simulink model "D53_LKAS_JLU_20200903_0931"  (R2018b)
settings: Solver=ode3  StartTime=0.0  StopTime=10.0  FixedStep=0.01  RelTol=1e-3  EnableMultiTasking=on
model workspace (MAT data in the model file):
  MCOS : class17 (value not decoded)
  MCOS : class17 (value not decoded)
  MCOS : class17 (value not decoded)
  MCOS : class17 (value not decoded)
  MCOS : class17 (value not decoded)
  MCOS : class17 (value not decoded)
  MCOS : class17 (value not decoded)
  MCOS : class17 (value not decoded)
  MCOS : class17 (value not decoded)
  MCOS : class17 (value not decoded)
  MCOS : class17 (value not decoded)
  MCOS : class17 (value not decoded)
  MCOS : class17 (value not decoded)
  MCOS : class17 (value not decoded)
  MCOS : class17 (value not decoded)
  MCOS : class17 (value not decoded)
  MCOS : class17 (value not decoded)
  MCOS : class17 (value not decoded)
  MCOS : class17 (value not decoded)
  MCOS : class17 (value not decoded)
  MCOS : class17 (value not decoded)
  MCOS : class17 (value not decoded)
  MCOS : class17 (value not decoded)
  MCOS : class17 (value not decoded)
  MCOS : class17 (value not decoded)
  MCOS : class17 (value not decoded)
  MCOS : class17 (value not decoded)
  MCOS : class17 (value not decoded)
  MCOS : class17 (value not decoded)
  MCOS : class17 (value not decoded)
  MCOS : class17 (value not decoded)
  MCOS : class17 (value not decoded)
  MCOS : class17 (value not decoded)
  MCOS : class17 (value not decoded)
  MCOS : class17 (value not decoded)
  MCOS : class17 (value not decoded)
  MCOS : class17 (value not decoded)
  MCOS : class17 (value not decoded)
  MCOS : class17 (value not decoded)
  MCOS : class17 (value not decoded)
  MCOS : class17 (value not decoded)
  MCOS : class17 (value not decoded)
  MCOS : class17 (value not decoded)
  MCOS : class17 (value not decoded)
  MCOS : class17 (value not decoded)
  MCOS : class17 (value not decoded)
  MCOS : class17 (value not decoded)
  MCOS : class17 (value not decoded)
  MCOS : class17 (value not decoded)
  MCOS : class17 (value not decoded)
  MCOS : class17 (value not decoded)
  MCOS : class17 (value not decoded)
  MCOS : class17 (value not decoded)
  MCOS : class17 (value not decoded)
  MCOS : class17 (value not decoded)
  MCOS : class17 (value not decoded)
  MCOS : class17 (value not decoded)
  MCOS : class17 (value not decoded)
  MCOS : class17 (value not decoded)
  MCOS : class17 (value not decoded)
  MCOS : class17 (value not decoded)
  MCOS : class17 (value not decoded)
  MCOS : class17 (value not decoded)
  MCOS : class17 (value not decoded)
  MCOS : class17 (value not decoded)
  MCOS : class17 (value not decoded)
  MCOS : class17 (value not decoded)
  MCOS : class17 (value not decoded)
  MCOS : class17 (value not decoded)
  MCOS : class17 (value not decoded)
  MCOS : class17 (value not decoded)
  MCOS : class17 (value not decoded)
  MCOS : class17 (value not decoded)
  MCOS : class17 (value not decoded)
  MCOS : class17 (value not decoded)
  MCOS : class17 (value not decoded)
  MCOS : class17 (value not decoded)
  MCOS : class17 (value not decoded)
  MCOS : class17 (value not decoded)
  MCOS : class17 (value not decoded)
  MCOS : class17 (value not decoded)
  MCOS : class17 (value not decoded)
  MCOS : class17 (value not decoded)
  MCOS : class17 (value not decoded)
  MCOS : class17 (value not decoded)
  MCOS : class17 (value not decoded)
  MCOS : class17 (value not decoded)
  MCOS : class17 (value not decoded)
  MCOS : class17 (value not decoded)
undefined symbols (not defined in the file): LKA_CarWidth, LKA_SampleTime, LKA_StrRatio_C, LKA_Veh2CamL_C, LKA_Veh2CamW_C, LKA_WhlBaseL_C, LL_CompSWA_C, LL_CrvtPrvwT_C, LL_DesDvt_C, LL_DvtComp_C, LL_DvtPrvwT_C, LL_DvtSpdDet_vDvtSpdMin_C, LL_HdAgExT_C, LL_HdAgPrvwT_C, LL_LAccMax_C, LL_LAccRMax_C, LL_LDW_EarliestWarnLine_C, LL_LDW_LatestWarnLine_C, LL_LDWS_SUPPRESS_HEADING, LL_LFClb_TFC_DiffCtlBalance, LL_LFClb_TFC_DiffCtrlMaxSWA, LL_LFClb_TFC_DiffCtrlRatio, LL_LFClb_TFC_facmGainLutGain1_C, LL_LFClb_TFC_facmGainLutGain2_C, LL_LFClb_TFC_facmIntegRatio, LL_LFClb_TFC_facmKlat_C, LL_LFClb_TFC_FfCtlRatio_C, LL_LFClb_TFC_phiIntegCtlMaxSWA_C, LL_LFClb_TFC_tiKlatPrvwT_C, LL_LFClb_TFC_vGainLutVehSpdLwr_C, LL_LFClb_TFC_vGainLutVehSpdUpr_C, LL_LKA_EarliestWarnLine_C, LL_LKA_LatestWarnLine_C, LL_LKAExPrcs_ExitC0Dvt, LL_LKAExPrcs_ExitC0Swt, LL_LKAExPrcs_tiExitTime1, LL_LKAExPrcs_tiExitTime2, LL_LKAExPrcs_tiExitTime3, LL_LKAS_OUT_OF_CONTROL_LAT_VEL, LL_LKAS_OUT_OF_CONTROL_TTLC, LL_LKASWASyn_M0, LL_LKASWASyn_M1, LL_LKASWASyn_M2, LL_LKASWASyn_M3K, LL_LKASWASyn_SWAaddMax, LL_LKASWASyn_T2, LL_LKASWASyn_tiTrqSwaRtTime, LL_LKASWASyn_tiTrqSwaTime, LL_LKASWASyn_TrqMax, LL_LKASWASyn_TrqSwaAddSwt, LL_LKASWASyn_TrqSwaRateDiff, LL_LSpdCompT_C, LL_lStpLngth_C, LL_MAX_DELAY_EPSSTAR_TIME, LL_MAX_DRIVER_TORQUE_DISABLE, LL_MAX_DRIVER_TORQUE_ENABLE, LL_MAX_LANE_WIDTH_DISABLE, LL_MAX_LANE_WIDTH_ENABLE, LL_MAX_LAT_ACC_DISABLE, LL_MAX_LAT_ACC_ENABLE ... (+30)
libraries: simulink x135, canmsglib x41, dspstat3 x3, simulink_extras x1
(part 6 of 18)

== system D53_LKAS_JLU_20200903_0931/SignalBusCreator/Subsystem3 ==
  Bus Creator20 : BusCreator  Inputs=10
  CAN Receive (CANRX) : S-Function  FunctionName=CAN_Rec_P  Parameters=uint8(Module-1),uint32(ID),uint8(Frameformat-1),uint8(Newflag),uint8(FIFO),double(sampletime)  SFunctionDeploymentMode=off  EnableBusSupport=off  mask(CAN_receive){Module=CAN_2, ID=1531, Frameformat=Extended (29-bit identifier), Newflag=off, FIFO=off, sampletime=0.01}
      mask prompts: Module "CAN Port:"; ID "CAN Frame ID:"; Frameformat "CAN Frame Format:"; FIFO "Overflow flag"
      mask init:
      | maskdisplay = canrecicon(Module,ID,Frameformat,Newflag,FIFO);
      | set_param(gcb, 'MaskDisplay', maskdisplay);
      mask TypeOptions Module: CAN_0 | CAN_1 | CAN_2 | CAN_3
      mask TypeOptions Frameformat: Standard (11-bit identifier) | Extended (29-bit identifier)
      mask Display: color('blue');text(0.98,0.9,'MPC5675K','horizontalAlignment','right');color('black');text(0.5,0.6,'FlexCAN_2 Receive','horizontalAlignment','center');text(0.5,0.35,'Extended ID:1531','horizontalAlignment','center');port_label('output',1,'CAN_Msg');
  CAN Receive (CANRX)1 : S-Function  FunctionName=CAN_Rec_P  Parameters=uint8(Module-1),uint32(ID),uint8(Frameformat-1),uint8(Newflag),uint8(FIFO),double(sampletime)  SFunctionDeploymentMode=off  EnableBusSupport=off  mask(CAN_receive){Module=CAN_2, ID=1523, Frameformat=Extended (29-bit identifier), Newflag=off, FIFO=off, sampletime=0.01}
      mask prompts: Module "CAN Port:"; ID "CAN Frame ID:"; Frameformat "CAN Frame Format:"; FIFO "Overflow flag"
      mask init:
      | maskdisplay = canrecicon(Module,ID,Frameformat,Newflag,FIFO);
      | set_param(gcb, 'MaskDisplay', maskdisplay);
      mask TypeOptions Module: CAN_0 | CAN_1 | CAN_2 | CAN_3
      mask TypeOptions Frameformat: Standard (11-bit identifier) | Extended (29-bit identifier)
      mask Display: color('blue');text(0.98,0.9,'MPC5675K','horizontalAlignment','right');color('black');text(0.5,0.6,'FlexCAN_2 Receive','horizontalAlignment','center');text(0.5,0.35,'Extended ID:1523','horizontalAlignment','center');port_label('output',1,'CAN_Msg');
  CAN Unpack1 : canmsglib/CAN Unpack  CANdbFile=D:\Work\02_LKA\LKAS\Documents\D53-SensorCAN.dbc  MsgList=Video_Lane_Next_Left_B  MsgName=Video_Lane_Next_Left_B  MsgIDType=Standard (11-bit identifier)  MsgIdentifier=1523  MsgLength=4  SignalInfo=Line_Width_5F3$17$7$2$2$1$0$1.000000e-02$0$0$1.270000e+00$#Me_Line_Changed_5F3$16$1$2$2$1$0$1$0$0$1$#TLC_5F3$8$8$2$2$1$0$1.000000e-02$0$0$2.550000e+00$#View_Range_5F3$0$8$2$2$1$0$5.000000e-01$0$0$1.275000e+02$#  NSignals=4  IDPort=off  TimestampPort=off  ErrorPort=off  RemotePort=off  LengthPort=off  StatusPort=off  StartBits=str2num('[int32(17);int32(16);int32(8);int32(0)]')  SignalSizes=str2num('[int32(7);int32(1);int32(8);int32(8)]')  ByteOrders=str2num('[int32(2);int32(2);int32(2);int32(2)]')  DataTypes=str2num('[int32(2);int32(2);int32(2);int32(2)]')  MultiplexTypes=str2num('[int32(1);int32(1);int32(1);int32(1)]')  MultiplexValues=str2num('[double(0);double(0);double(0);double(0)]')  Factors=str2num('[double(1.000000e-02);double(1);double(1.000000e-02);double(5.000000e-01)]')  Offsets=str2num('[double(0);double(0);double(0);double(0)]')  Minimums=str2num('[double(0);double(0);double(0);double(0)]')  Maximums=str2num('[double(1.270000e+00);double(1);double(2.550000e+00);double(1.275000e+02)]')  ApplyMinMax=off
      settings: SourceProductName=Simulink Real-Time  SourceProductBaseCode=XP  DataFormat=CANdb specified signals
  CAN Unpack13 : canmsglib/CAN Unpack  CANdbFile=D:\Work\02_LKA\LKAS\Documents\D53-SensorCAN.dbc  MsgList=Video_Lane_Next_Left_A  MsgName=Video_Lane_Next_Left_A  MsgIDType=Standard (11-bit identifier)  MsgIdentifier=1531  MsgLength=8  SignalInfo=C0_5FB$44$12$2$1$1$0$1.000000e-02$0$-2.048000e+01$2.047000e+01$#C1_5FB$50$10$2$1$1$0$9.765625e-04$0$-3.570000e-01$3.570000e-01$#C2_5FB$24$16$2$1$1$0$1.000000e-06$0$-3.276800e-02$3.276600e-02$#C3_5FB$8$16$2$1$1$0$4.000000e-09$0$-1.310720e-04$1.310680e-04$#Line_Type_5FB$59$3$2$2$1$0$1$0$0$7$#Quality_5FB$62$2$2$2$1$0$1$0$0$3$#  NSignals=6  IDPort=off  TimestampPort=off  ErrorPort=off  RemotePort=off  LengthPort=off  StatusPort=off  StartBits=str2num('[int32(44);int32(50);int32(24);int32(8);int32(59);int32(62)]')  SignalSizes=str2num('[int32(12);int32(10);int32(16);int32(16);int32(3);int32(2)]')  ByteOrders=str2num('[int32(2);int32(2);int32(2);int32(2);int32(2);int32(2)]')  DataTypes=str2num('[int32(1);int32(1);int32(1);int32(1);int32(2);int32(2)]')  MultiplexTypes=str2num('[int32(1);int32(1);int32(1);int32(1);int32(1);int32(1)]')  MultiplexValues=str2num('[double(0);double(0);double(0);double(0);double(0);double(0)]')  Factors=str2num('[double(1.000000e-02);double(9.765625e-04);double(1.000000e-06);double(4.000000e-09);double(1);double(1)]')  Offsets=str2num('[double(0);double(0);double(0);double(0);double(0);double(0)]')  Minimums=str2num('[double(-2.048000e+01);double(-3.570000e-01);double(-3.276800e-02);double(-1.310720e-04);double(0);double(0)]')  Maximums=str2num('[double(2.047000e+01);double(3.570000e-01);double(3.276600e-02);double(1.310680e-04);double(7);double(3)]')  ApplyMinMax=off
      settings: SourceProductName=Simulink Real-Time  SourceProductBaseCode=XP  DataFormat=CANdb specified signals
  Data Type Conversion{,1..3,5..6,9} (7 alike) : DataTypeConversion  OutDataTypeStr=single
  Data Type Conversion4 : DataTypeConversion  OutDataTypeStr=uint8
  Data Type Conversion7 : DataTypeConversion  OutDataTypeStr=uint8
  Data Type Conversion8 : DataTypeConversion  OutDataTypeStr=uint8
  bsOriL1Info : Outport
  wires:
  CAN Receive (CANRX)/1 -> CAN Unpack13/1
  Data Type Conversion/1 -> Bus Creator20/4  "O_L1_C0"
  CAN Unpack13/4 -> Data Type Conversion3/1
  CAN Unpack13/5 -> Data Type Conversion7/1
  Data Type Conversion6/1 -> Bus Creator20/9  "O_L1_W"
  CAN Unpack13/2 -> Data Type Conversion1/1
  CAN Unpack1/4 -> Data Type Conversion5/1
  Data Type Conversion4/1 -> Bus Creator20/5  "O_L1_Q"
  CAN Unpack1/2 -> Data Type Conversion8/1
  CAN Unpack13/6 -> Data Type Conversion4/1
  CAN Unpack13/1 -> Data Type Conversion/1
  CAN Unpack1/1 -> Data Type Conversion6/1
  CAN Unpack1/3 -> Data Type Conversion9/1
  CAN Unpack13/3 -> Data Type Conversion2/1
  Data Type Conversion9/1 -> Bus Creator20/8  "O_L1_TLC"
  Data Type Conversion7/1 -> Bus Creator20/6  "O_L1_Type"
  Bus Creator20/1 -> bsOriL1Info/1  "bsOriL1Info"
  Data Type Conversion5/1 -> Bus Creator20/7  "O_L1_VR"
  Data Type Conversion3/1 -> Bus Creator20/1  "O_L1_C3"
  Data Type Conversion8/1 -> Bus Creator20/10  "O_L1_LC"
  Data Type Conversion1/1 -> Bus Creator20/3  "O_L1_C1"
  Data Type Conversion2/1 -> Bus Creator20/2  "O_L1_C2"
  CAN Receive (CANRX)1/1 -> CAN Unpack1/1

== system D53_LKAS_JLU_20200903_0931/SignalBusCreator/Subsystem4 ==
  Bus Creator22 : BusCreator  Inputs=10
  CAN Receive (CANRX) : S-Function  FunctionName=CAN_Rec_P  Parameters=uint8(Module-1),uint32(ID),uint8(Frameformat-1),uint8(Newflag),uint8(FIFO),double(sampletime)  SFunctionDeploymentMode=off  EnableBusSupport=off  mask(CAN_receive){Module=CAN_2, ID=1534, Frameformat=Extended (29-bit identifier), Newflag=off, FIFO=off, sampletime=0.01}
      mask prompts: Module "CAN Port:"; ID "CAN Frame ID:"; Frameformat "CAN Frame Format:"; FIFO "Overflow flag"
      mask init:
      | maskdisplay = canrecicon(Module,ID,Frameformat,Newflag,FIFO);
      | set_param(gcb, 'MaskDisplay', maskdisplay);
      mask TypeOptions Module: CAN_0 | CAN_1 | CAN_2 | CAN_3
      mask TypeOptions Frameformat: Standard (11-bit identifier) | Extended (29-bit identifier)
      mask Display: color('blue');text(0.98,0.9,'MPC5675K','horizontalAlignment','right');color('black');text(0.5,0.6,'FlexCAN_2 Receive','horizontalAlignment','center');text(0.5,0.35,'Extended ID:1534','horizontalAlignment','center');port_label('output',1,'CAN_Msg');
  CAN Receive (CANRX)1 : S-Function  FunctionName=CAN_Rec_P  Parameters=uint8(Module-1),uint32(ID),uint8(Frameformat-1),uint8(Newflag),uint8(FIFO),double(sampletime)  SFunctionDeploymentMode=off  EnableBusSupport=off  mask(CAN_receive){Module=CAN_2, ID=1524, Frameformat=Extended (29-bit identifier), Newflag=off, FIFO=off, sampletime=0.01}
      mask prompts: Module "CAN Port:"; ID "CAN Frame ID:"; Frameformat "CAN Frame Format:"; FIFO "Overflow flag"
      mask init:
      | maskdisplay = canrecicon(Module,ID,Frameformat,Newflag,FIFO);
      | set_param(gcb, 'MaskDisplay', maskdisplay);
      mask TypeOptions Module: CAN_0 | CAN_1 | CAN_2 | CAN_3
      mask TypeOptions Frameformat: Standard (11-bit identifier) | Extended (29-bit identifier)
      mask Display: color('blue');text(0.98,0.9,'MPC5675K','horizontalAlignment','right');color('black');text(0.5,0.6,'FlexCAN_2 Receive','horizontalAlignment','center');text(0.5,0.35,'Extended ID:1524','horizontalAlignment','center');port_label('output',1,'CAN_Msg');
  CAN Unpack1 : canmsglib/CAN Unpack  CANdbFile=D:\Work\02_LKA\LKAS\Documents\D53-SensorCAN.dbc  MsgList=Video_Lane_Next_Right_B  MsgName=Video_Lane_Next_Right_B  MsgIDType=Standard (11-bit identifier)  MsgIdentifier=1524  MsgLength=4  SignalInfo=Line_Width_5F4$17$7$2$2$1$0$1.000000e-02$0$0$1.270000e+00$#Me_Line_Changed_5F4$16$1$2$2$1$0$1$0$0$1$#TLC_5F4$8$8$2$2$1$0$1.000000e-02$0$0$2.550000e+00$#View_Range_5F4$0$8$2$2$1$0$5.000000e-01$0$0$1.275000e+02$#  NSignals=4  IDPort=off  TimestampPort=off  ErrorPort=off  RemotePort=off  LengthPort=off  StatusPort=off  StartBits=str2num('[int32(17);int32(16);int32(8);int32(0)]')  SignalSizes=str2num('[int32(7);int32(1);int32(8);int32(8)]')  ByteOrders=str2num('[int32(2);int32(2);int32(2);int32(2)]')  DataTypes=str2num('[int32(2);int32(2);int32(2);int32(2)]')  MultiplexTypes=str2num('[int32(1);int32(1);int32(1);int32(1)]')  MultiplexValues=str2num('[double(0);double(0);double(0);double(0)]')  Factors=str2num('[double(1.000000e-02);double(1);double(1.000000e-02);double(5.000000e-01)]')  Offsets=str2num('[double(0);double(0);double(0);double(0)]')  Minimums=str2num('[double(0);double(0);double(0);double(0)]')  Maximums=str2num('[double(1.270000e+00);double(1);double(2.550000e+00);double(1.275000e+02)]')  ApplyMinMax=off
      settings: SourceProductName=Simulink Real-Time  SourceProductBaseCode=XP  DataFormat=CANdb specified signals
  CAN Unpack13 : canmsglib/CAN Unpack  CANdbFile=D:\Work\02_LKA\LKAS\Documents\D53-SensorCAN.dbc  MsgList=Video_Lane_Next_Right_A  MsgName=Video_Lane_Next_Right_A  MsgIDType=Standard (11-bit identifier)  MsgIdentifier=1534  MsgLength=8  SignalInfo=C0_5FE$44$12$2$1$1$0$1.000000e-02$0$-2.048000e+01$2.047000e+01$#C1_5FE$50$10$2$1$1$0$9.765625e-04$0$-3.570000e-01$3.570000e-01$#C2_5FE$24$16$2$1$1$0$1.000000e-06$0$-3.276800e-02$3.276600e-02$#C3_5FE$8$16$2$1$1$0$4.000000e-09$0$-1.310720e-04$1.310680e-04$#Line_Type_5FE$59$3$2$2$1$0$1$0$0$7$#Quality_5FE$62$2$2$2$1$0$1$0$0$3$#  NSignals=6  IDPort=off  TimestampPort=off  ErrorPort=off  RemotePort=off  LengthPort=off  StatusPort=off  StartBits=str2num('[int32(44);int32(50);int32(24);int32(8);int32(59);int32(62)]')  SignalSizes=str2num('[int32(12);int32(10);int32(16);int32(16);int32(3);int32(2)]')  ByteOrders=str2num('[int32(2);int32(2);int32(2);int32(2);int32(2);int32(2)]')  DataTypes=str2num('[int32(1);int32(1);int32(1);int32(1);int32(2);int32(2)]')  MultiplexTypes=str2num('[int32(1);int32(1);int32(1);int32(1);int32(1);int32(1)]')  MultiplexValues=str2num('[double(0);double(0);double(0);double(0);double(0);double(0)]')  Factors=str2num('[double(1.000000e-02);double(9.765625e-04);double(1.000000e-06);double(4.000000e-09);double(1);double(1)]')  Offsets=str2num('[double(0);double(0);double(0);double(0);double(0);double(0)]')  Minimums=str2num('[double(-2.048000e+01);double(-3.570000e-01);double(-3.276800e-02);double(-1.310720e-04);double(0);double(0)]')  Maximums=str2num('[double(2.047000e+01);double(3.570000e-01);double(3.276600e-02);double(1.310680e-04);double(7);double(3)]')  ApplyMinMax=off
      settings: SourceProductName=Simulink Real-Time  SourceProductBaseCode=XP  DataFormat=CANdb specified signals
  Data Type Conversion{,6..8,10..11,14} (7 alike) : DataTypeConversion  OutDataTypeStr=single
  Data Type Conversion12 : DataTypeConversion  OutDataTypeStr=uint8
  Data Type Conversion13 : DataTypeConversion  OutDataTypeStr=uint8
  Data Type Conversion9 : DataTypeConversion  OutDataTypeStr=uint8
  bsOriR1Info : Outport
  wires:
  Data Type Conversion6/1 -> Bus Creator22/3  "O_R1_C1"
  Data Type Conversion11/1 -> Bus Creator22/9  "O_R1_W"
  Data Type Conversion14/1 -> Bus Creator22/8  "O_R1_TLC"
  Data Type Conversion/1 -> Bus Creator22/4  "O_R1_C0"
  Data Type Conversion7/1 -> Bus Creator22/2  "O_R1_C2"
  Data Type Conversion9/1 -> Bus Creator22/5  "O_R1_Q"
  Data Type Conversion13/1 -> Bus Creator22/10  "O_R1_LC"
  Data Type Conversion8/1 -> Bus Creator22/1  "O_R1_C3"
  CAN Unpack13/2 -> Data Type Conversion6/1
  CAN Unpack13/3 -> Data Type Conversion7/1
  Data Type Conversion12/1 -> Bus Creator22/6  "O_R1_Type"
  Data Type Conversion10/1 -> Bus Creator22/7  "O_R1_VR"
  CAN Unpack13/1 -> Data Type Conversion/1
  CAN Unpack1/4 -> Data Type Conversion10/1
  CAN Receive (CANRX)/1 -> CAN Unpack13/1
  CAN Unpack1/3 -> Data Type Conversion14/1
  CAN Unpack13/5 -> Data Type Conversion12/1
  CAN Unpack13/6 -> Data Type Conversion9/1
  CAN Unpack1/2 -> Data Type Conversion13/1
  CAN Unpack1/1 -> Data Type Conversion11/1
  CAN Unpack13/4 -> Data Type Conversion8/1
  Bus Creator22/1 -> bsOriR1Info/1  "bsOriR1Info"
  CAN Receive (CANRX)1/1 -> CAN Unpack1/1

== system D53_LKAS_JLU_20200903_0931/SignalBusCreator/Subsystem5 ==
  Bus Creator3 : BusCreator  Inputs=4
  CAN Recv (CANRx]) : S-Function  FunctionName=CAN_Rec_P  Parameters=uint8(Module-1),uint32(ID),uint8(Frameformat-1),uint8(Newflag),uint8(FIFO),double(sampletime)  SFunctionDeploymentMode=off  EnableBusSupport=off  mask(CAN_receive){Module=CAN_1, ID=773, Frameformat=Standard (11-bit identifier), Newflag=off, FIFO=off, sampletime=0.01}
      mask prompts: Module "CAN Port:"; ID "CAN Frame ID:"; Frameformat "CAN Frame Format:"; FIFO "Overflow flag"
      mask init:
      | maskdisplay = canrecicon(Module,ID,Frameformat,Newflag,FIFO);
      | set_param(gcb, 'MaskDisplay', maskdisplay);
      mask TypeOptions Module: CAN_0 | CAN_1 | CAN_2 | CAN_3
      mask TypeOptions Frameformat: Standard (11-bit identifier) | Extended (29-bit identifier)
      mask Display: color('blue');text(0.98,0.9,'MPC5675K','horizontalAlignment','right');color('black');text(0.5,0.6,'FlexCAN_1 Receive','horizontalAlignment','center');text(0.5,0.35,'Standard ID:773','horizontalAlignment','center');port_label('output',1,'CAN_Msg');
  CAN Unpack1 : canmsglib/CAN Unpack  CANdbFile=D:\Work\02_LKA\LKAS\Documents\D53-PSA1CAN.dbc  MsgList=EPS_305_PSA1  MsgName=EPS_305_PSA1  MsgIDType=Standard (11-bit identifier)  MsgIdentifier=773  MsgLength=7  SignalInfo=Absolute_Steering_Wheel_angle$54$1$2$2$1$0$1$0$-Inf$Inf$#Initialization_steering_angle$55$1$2$2$1$0$1$0$-Inf$Inf$#Internal_SWS_status$24$1$2$2$1$0$1$0$-Inf$Inf$#SWS_calibration$25$1$2$2$1$0$1$0$-Inf$Inf$#SWS_checksum$36$4$2$2$1$0$1$0$-Inf$Inf$#SWS_fault_code$27$4$2$2$1$0$1$0$-Inf$Inf$#SWS_trim$26$1$2$2$1$0$1$0$-Inf$Inf$#Steering_wheel_angle$8$16$2$1$1$0$1.000000e-01$0$-780$780$#Steering_wheel_rotation_speed$16$8$2$2$1$0$4$0$0$1016$#Steering_wheel_sensor_direction$31$1$2$2$1$0$1$0$-Inf$Inf$#bits_Compute_counter_for_SWS$32$4$2$2$1$0$1$0$0$15$#indication_of_steering_wheel$52$2$2$2$1$0$1$0$-Inf$Inf$#  NSignals=12  IDPort=off  TimestampPort=off  ErrorPort=off  RemotePort=off  LengthPort=off  StatusPort=off  StartBits=str2num('[int32(54);int32(55);int32(24);int32(25);int32(36);int32(27);int32(26);int32(8);int32(16);int32(31);int32(32);int32(52)]')  SignalSizes=str2num('[int32(1);int32(1);int32(1);int32(1);int32(4);int32(4);int32(1);int32(16);int32(8);int32(1);int32(4);int32(2)]')  ByteOrders=str2num('[int32(2);int32(2);int32(2);int32(2);int32(2);int32(2);int32(2);int32(2);int32(2);int32(2);int32(2);int32(2)]')  DataTypes=str2num('[int32(2);int32(2);int32(2);int32(2);int32(2);int32(2);int32(2);int32(1);int32(2);int32(2);int32(2);int32(2)]')  MultiplexTypes=str2num('[int32(1);int32(1);int32(1);int32(1);int32(1);int32(1);int32(1);int32(1);int32(1);int32(1);int32(1);int32(1)]')  MultiplexValues=str2num('[double(0);double(0);double(0);double(0);double(0);double(0);double(0);double(0);double(0);double(0);double(0);double(0)]')  Factors=str2num('[double(1);double(1);double(1);double(1);double(1);double(1);double(1);double(1.000000e-01);double(4);double(1);double(1);double(1)]')  Offsets=str2num('[double(0);double(0);double(0);double(0);double(0);double(0);double(0);double(0);double(0);double(0);double(0);double(0)]')  Minimums=str2num('[double(-Inf);double(-Inf);double(-Inf);double(-Inf);double(-Inf);double(-Inf);double(-Inf);double(-780);double(0);double(-Inf);double(0);double(-Inf)]')  Maximums=str2num('[double(Inf);double(Inf);double(Inf);double(Inf);double(Inf);double(Inf);double(Inf);double(780);double(1016);double(Inf);double(15);double(Inf)]')  ApplyMinMax=off
      settings: SourceProductName=Simulink Real-Time  SourceProductBaseCode=XP  DataFormat=CANdb specified signals
  Data Type Conversion1 : DataTypeConversion  OutDataTypeStr=single
  Data Type Conversion2 : DataTypeConversion  OutDataTypeStr=single
  Data Type Conversion46 : DataTypeConversion  OutDataTypeStr=uint8
  Data Type Conversion47 : DataTypeConversion  OutDataTypeStr=uint8
  Terminator{1..8} (8 alike) : Terminator
  bsSWAInfo : Outport
  wires:
  Data Type Conversion46/1 -> Bus Creator3/3  "SWS_Fault_Code"
  CAN Unpack1/4 -> Terminator3/1
  CAN Unpack1/5 -> Terminator4/1
  CAN Unpack1/11 -> Terminator7/1
  Bus Creator3/1 -> bsSWAInfo/1  "bsSWAInfo"
  CAN Unpack1/12 -> Terminator8/1
  CAN Unpack1/8 -> Data Type Conversion1/1  "SWARx_phiSWA"
  CAN Unpack1/2 -> Terminator2/1  "SWARx_phiSWA"
  CAN Unpack1/9 -> Data Type Conversion2/1  "SW_Angle_Speed"
  CAN Unpack1/10 -> Terminator6/1
  CAN Unpack1/6 -> Data Type Conversion46/1
  CAN Unpack1/3 -> Data Type Conversion47/1
  CAN Recv (CANRx])/1 -> CAN Unpack1/1
  Data Type Conversion47/1 -> Bus Creator3/4  "SAS_In_Status"
  CAN Unpack1/1 -> Terminator1/1
  CAN Unpack1/7 -> Terminator5/1
  Data Type Conversion1/1 -> Bus Creator3/1  "SW_Angle"
  Data Type Conversion2/1 -> Bus Creator3/2  "SW_Angle_Speed"

== system D53_LKAS_JLU_20200903_0931/SignalBusCreator/Subsystem6 ==
  Bus Creator2 : BusCreator  Inputs=9
  CAN Recv : S-Function  FunctionName=CAN_Rec_P  Parameters=uint8(Module-1),uint32(ID),uint8(Frameformat-1),uint8(Newflag),uint8(FIFO),double(sampletime)  SFunctionDeploymentMode=off  EnableBusSupport=off  mask(CAN_receive){Module=CAN_1, ID=1173, Frameformat=Standard (11-bit identifier), Newflag=off, FIFO=off, sampletime=0.01}
      mask prompts: Module "CAN Port:"; ID "CAN Frame ID:"; Frameformat "CAN Frame Format:"; FIFO "Overflow flag"
      mask init:
      | maskdisplay = canrecicon(Module,ID,Frameformat,Newflag,FIFO);
      | set_param(gcb, 'MaskDisplay', maskdisplay);
      mask TypeOptions Module: CAN_0 | CAN_1 | CAN_2 | CAN_3
      mask TypeOptions Frameformat: Standard (11-bit identifier) | Extended (29-bit identifier)
      mask Display: color('blue');text(0.98,0.9,'MPC5675K','horizontalAlignment','right');color('black');text(0.5,0.6,'FlexCAN_1 Receive','horizontalAlignment','center');text(0.5,0.35,'Standard ID:1173','horizontalAlignment','center');port_label('output',1,'CAN_Msg');
  CAN Unpack : canmsglib/CAN Unpack  CANdbFile=D:\Work\02_LKA\LKAS\Documents\D53-PSA1CAN.dbc  MsgList=EPS_495_PSA1  MsgName=EPS_495_PSA1  MsgIDType=Standard (11-bit identifier)  MsgIdentifier=1173  MsgLength=4  SignalInfo=Power_steering_status$14$2$2$2$1$0$1$0$-Inf$Inf$#State_indicating_steering_or_not$17$1$2$2$1$0$1$0$-Inf$Inf$#State_of_EPS_for_LKA_function$18$3$2$2$1$0$1$0$-Inf$Inf$#Steering_wheel_torque$0$8$2$1$1$0$2.500000e-01$0$-32$3.150000e+01$#Torque_limitation_if_DAE_limit$16$1$2$2$1$0$1$0$-Inf$Inf$#  NSignals=5  IDPort=off  TimestampPort=off  ErrorPort=off  RemotePort=off  LengthPort=off  StatusPort=off  StartBits=str2num('[int32(14);int32(17);int32(18);int32(0);int32(16)]')  SignalSizes=str2num('[int32(2);int32(1);int32(3);int32(8);int32(1)]')  ByteOrders=str2num('[int32(2);int32(2);int32(2);int32(2);int32(2)]')  DataTypes=str2num('[int32(2);int32(2);int32(2);int32(1);int32(2)]')  MultiplexTypes=str2num('[int32(1);int32(1);int32(1);int32(1);int32(1)]')  MultiplexValues=str2num('[double(0);double(0);double(0);double(0);double(0)]')  Factors=str2num('[double(1);double(1);double(1);double(2.500000e-01);double(1)]')  Offsets=str2num('[double(0);double(0);double(0);double(0);double(0)]')  Minimums=str2num('[double(-Inf);double(-Inf);double(-Inf);double(-32);double(-Inf)]')  Maximums=str2num('[double(Inf);double(Inf);double(Inf);double(3.150000e+01);double(Inf)]')  ApplyMinMax=off
      settings: SourceProductName=Simulink Real-Time  SourceProductBaseCode=XP  DataFormat=CANdb specified signals
  Data Type Conversion : DataTypeConversion  OutDataTypeStr=uint8
  Data Type Conversion1 : DataTypeConversion  OutDataTypeStr=single
  Data Type Conversion2 : DataTypeConversion  OutDataTypeStr=uint8
  Data Type Conversion3 : DataTypeConversion  OutDataTypeStr=uint8
  Ground{,1..4} (5 alike) : Ground
  Terminator : Terminator
  bsEPSInfo : Outport
  wires:
  Data Type Conversion/1 -> Bus Creator2/1  "EPS_LKA_State"
  CAN Unpack/3 -> Data Type Conversion/1
  Ground/1 -> Bus Creator2/4  "EPS_Trq_State"
  Ground4/1 -> Bus Creator2/8  "EPS_LKA_Current"
  Data Type Conversion2/1 -> Bus Creator2/3  "EPS_Error_State"
  CAN Unpack/1 -> Data Type Conversion2/1
  CAN Recv/1 -> CAN Unpack/1
  Ground3/1 -> Bus Creator2/7  "EPS_TrqLim_State"
  Data Type Conversion1/1 -> Bus Creator2/2  "EPS_SW_Trq"
  Data Type Conversion3/1 -> Bus Creator2/9  "EPS_SWHold_State"
  CAN Unpack/4 -> Data Type Conversion1/1
  CAN Unpack/2 -> Data Type Conversion3/1
  Ground2/1 -> Bus Creator2/6  "SAS_Trim_State"
  CAN Unpack/5 -> Terminator/1
  Ground1/1 -> Bus Creator2/5  "SAS_Clb_State"
  Bus Creator2/1 -> bsEPSInfo/1  "bsEPSInfo"

== system D53_LKAS_JLU_20200903_0931/SignalBusCreator/Subsystem7 ==
  Bus Creator18 : BusCreator  Inputs=3
  CAN Recv : S-Function  FunctionName=CAN_Rec_P  Parameters=uint8(Module-1),uint32(ID),uint8(Frameformat-1),uint8(Newflag),uint8(FIFO),double(sampletime)  SFunctionDeploymentMode=off  EnableBusSupport=off  mask(CAN_receive){Module=CAN_2, ID=1110, Frameformat=Standard (11-bit identifier), Newflag=off, FIFO=off, sampletime=0.05}
      mask prompts: Module "CAN Port:"; ID "CAN Frame ID:"; Frameformat "CAN Frame Format:"; FIFO "Overflow flag"
      mask init:
      | maskdisplay = canrecicon(Module,ID,Frameformat,Newflag,FIFO);
      | set_param(gcb, 'MaskDisplay', maskdisplay);
      mask TypeOptions Module: CAN_0 | CAN_1 | CAN_2 | CAN_3
      mask TypeOptions Frameformat: Standard (11-bit identifier) | Extended (29-bit identifier)
      mask Display: color('blue');text(0.98,0.9,'MPC5675K','horizontalAlignment','right');color('black');text(0.5,0.6,'FlexCAN_2 Receive','horizontalAlignment','center');text(0.5,0.35,'Standard ID:1110','horizontalAlignment','center');port_label('output',1,'CAN_Msg');
  CAN Unpack : canmsglib/CAN Unpack  CANdbFile=D:\Work\02_LKA\LKAS\Documents\D53-SensorCAN.dbc  MsgList=Video_Lane_Header  MsgName=Video_Lane_Header  MsgIDType=Standard (11-bit identifier)  MsgIdentifier=1110  MsgLength=1  SignalInfo=Construction_Area$6$1$2$2$1$0$1$0$0$1$#LaneModuleValid$7$1$2$2$1$0$1$0$0$1$#Road_Type$4$2$2$2$1$0$1$0$0$3$#  NSignals=3  IDPort=off  TimestampPort=off  ErrorPort=off  RemotePort=off  LengthPort=off  StatusPort=off  StartBits=str2num('[int32(6);int32(7);int32(4)]')  SignalSizes=str2num('[int32(1);int32(1);int32(2)]')  ByteOrders=str2num('[int32(2);int32(2);int32(2)]')  DataTypes=str2num('[int32(2);int32(2);int32(2)]')  MultiplexTypes=str2num('[int32(1);int32(1);int32(1)]')  MultiplexValues=str2num('[double(0);double(0);double(0)]')  Factors=str2num('[double(1);double(1);double(1)]')  Offsets=str2num('[double(0);double(0);double(0)]')  Minimums=str2num('[double(0);double(0);double(0)]')  Maximums=str2num('[double(1);double(1);double(3)]')  ApplyMinMax=off
      settings: SourceProductName=Simulink Real-Time  SourceProductBaseCode=XP  DataFormat=CANdb specified signals
  Data Type Conversion : DataTypeConversion  OutDataTypeStr=uint8
  Data Type Conversion1 : DataTypeConversion  OutDataTypeStr=uint8
  Data Type Conversion2 : DataTypeConversion  OutDataTypeStr=uint8
  bsOriLaneInfo : Outport
  wires:
  CAN Unpack/3 -> Data Type Conversion2/1  "O_Lane_RoadType"
  CAN Unpack/2 -> Data Type Conversion1/1  "O_Lane_Valid"
  CAN Recv/1 -> CAN Unpack/1
  CAN Unpack/1 -> Data Type Conversion/1  "O_Lane_ConsArea"
  Bus Creator18/1 -> bsOriLaneInfo/1  "bsOriLaneInfo"
  Data Type Conversion/1 -> Bus Creator18/2  "O_Lane_ConsArea"
  Data Type Conversion1/1 -> Bus Creator18/1  "O_Lane_Valid"
  Data Type Conversion2/1 -> Bus Creator18/3  "O_Lane_RoadType"

== system D53_LKAS_JLU_20200903_0931/SignalBusCreator/Subsystem8 ==
  Bus Creator9 : BusCreator  Inputs=10
  CAN Recv (CANRx]) : S-Function  FunctionName=CAN_Rec_P  Parameters=uint8(Module-1),uint32(ID),uint8(Frameformat-1),uint8(Newflag),uint8(FIFO),double(sampletime)  SFunctionDeploymentMode=off  EnableBusSupport=off  mask(CAN_receive){Module=CAN_1, ID=973, Frameformat=Standard (11-bit identifier), Newflag=off, FIFO=off, sampletime=0.01}
      mask prompts: Module "CAN Port:"; ID "CAN Frame ID:"; Frameformat "CAN Frame Format:"; FIFO "Overflow flag"
      mask init:
      | maskdisplay = canrecicon(Module,ID,Frameformat,Newflag,FIFO);
      | set_param(gcb, 'MaskDisplay', maskdisplay);
      mask TypeOptions Module: CAN_0 | CAN_1 | CAN_2 | CAN_3
      mask TypeOptions Frameformat: Standard (11-bit identifier) | Extended (29-bit identifier)
      mask Display: color('blue');text(0.98,0.9,'MPC5675K','horizontalAlignment','right');color('black');text(0.5,0.6,'FlexCAN_1 Receive','horizontalAlignment','center');text(0.5,0.35,'Standard ID:973','horizontalAlignment','center');port_label('output',1,'CAN_Msg');
  CAN Recv (CANRx])1 : S-Function  FunctionName=CAN_Rec_P  Parameters=uint8(Module-1),uint32(ID),uint8(Frameformat-1),uint8(Newflag),uint8(FIFO),double(sampletime)  SFunctionDeploymentMode=off  EnableBusSupport=off  mask(CAN_receive){Module=CAN_1, ID=909, Frameformat=Extended (29-bit identifier), Newflag=off, FIFO=off, sampletime=0.04}
      mask prompts: Module "CAN Port:"; ID "CAN Frame ID:"; Frameformat "CAN Frame Format:"; FIFO "Overflow flag"
      mask init:
      | maskdisplay = canrecicon(Module,ID,Frameformat,Newflag,FIFO);
      | set_param(gcb, 'MaskDisplay', maskdisplay);
      mask TypeOptions Module: CAN_0 | CAN_1 | CAN_2 | CAN_3
      mask TypeOptions Frameformat: Standard (11-bit identifier) | Extended (29-bit identifier)
      mask Display: color('blue');text(0.98,0.9,'MPC5675K','horizontalAlignment','right');color('black');text(0.5,0.6,'FlexCAN_1 Receive','horizontalAlignment','center');text(0.5,0.35,'Extended ID:909','horizontalAlignment','center');port_label('output',1,'CAN_Msg');
  CAN Unpack : canmsglib/CAN Unpack  CANdbFile=D:\Work\02_LKA\LKAS\Documents\D53-PSA1CAN.dbc  MsgList=ESC_3CD_PSA1  MsgName=ESC_3CD_PSA1  MsgIDType=Standard (11-bit identifier)  MsgIdentifier=973  MsgLength=8  SignalInfo=Brake_pedal_disabled_UC_Brake$37$1$2$2$1$0$1$0$-Inf$Inf$#Frame_checksum3CD$60$4$2$2$1$0$1$0$-Inf$Inf$#Lateral_acceleration$8$16$2$1$1$0$5.000000e-02$0$-15$15$#TMC_pressure$52$12$2$2$1$0$1.000000e-01$-55$-55$3.544000e+02$#Yaw_speed$24$16$2$1$1$0$1.000000e-01$0$-100$100$#bits_compute_process_counter3CD$56$4$2$2$1$0$1$0$0$15$#  NSignals=6  IDPort=off  TimestampPort=off  ErrorPort=off  RemotePort=off  LengthPort=off  StatusPort=off  StartBits=str2num('[int32(37);int32(60);int32(8);int32(52);int32(24);int32(56)]')  SignalSizes=str2num('[int32(1);int32(4);int32(16);int32(12);int32(16);int32(4)]')  ByteOrders=str2num('[int32(2);int32(2);int32(2);int32(2);int32(2);int32(2)]')  DataTypes=str2num('[int32(2);int32(2);int32(1);int32(2);int32(1);int32(2)]')  MultiplexTypes=str2num('[int32(1);int32(1);int32(1);int32(1);int32(1);int32(1)]')  MultiplexValues=str2num('[double(0);double(0);double(0);double(0);double(0);double(0)]')  Factors=str2num('[double(1);double(1);double(5.000000e-02);double(1.000000e-01);double(1.000000e-01);double(1)]')  Offsets=str2num('[double(0);double(0);double(0);double(-55);double(0);double(0)]')  Minimums=str2num('[double(-Inf);double(-Inf);double(-15);double(-55);double(-100);double(0)]')  Maximums=str2num('[double(Inf);double(Inf);double(15);double(3.544000e+02);double(100);double(15)]')  ApplyMinMax=off
      settings: SourceProductName=Simulink Real-Time  SourceProductBaseCode=XP  DataFormat=CANdb specified signals
  CAN Unpack1 : canmsglib/CAN Unpack  CANdbFile=D:\Work\02_LKA\LKAS\Documents\D53-PSA1CAN.dbc  MsgList=ESC_38D_PSA1  MsgName=ESC_38D_PSA1  MsgIDType=Standard (11-bit identifier)  MsgIdentifier=909  MsgLength=8  SignalInfo=ABR_dynamic_checksum$40$4$2$2$1$0$1$0$-Inf$Inf$#Vehicle_driving_direction$52$2$2$2$1$0$1$0$-Inf$Inf$#Vehicle_speed_of_wheelsensor$8$16$2$2$1$0$1.000000e-02$0$0$6.553400e+02$#Vehiclespeed_unavailability_flag$50$2$2$2$1$0$1$0$-Inf$Inf$#bits_compute_for_UC_brake$44$4$2$2$1$0$1$0$0$15$#  NSignals=5  IDPort=off  TimestampPort=off  ErrorPort=off  RemotePort=off  LengthPort=off  StatusPort=off  StartBits=str2num('[int32(40);int32(52);int32(8);int32(50);int32(44)]')  SignalSizes=str2num('[int32(4);int32(2);int32(16);int32(2);int32(4)]')  ByteOrders=str2num('[int32(2);int32(2);int32(2);int32(2);int32(2)]')  DataTypes=str2num('[int32(2);int32(2);int32(2);int32(2);int32(2)]')  MultiplexTypes=str2num('[int32(1);int32(1);int32(1);int32(1);int32(1)]')  MultiplexValues=str2num('[double(0);double(0);double(0);double(0);double(0)]')  Factors=str2num('[double(1);double(1);double(1.000000e-02);double(1);double(1)]')  Offsets=str2num('[double(0);double(0);double(0);double(0);double(0)]')  Minimums=str2num('[double(-Inf);double(-Inf);double(0);double(-Inf);double(0)]')  Maximums=str2num('[double(Inf);double(Inf);double(6.553400e+02);double(Inf);double(15)]')  ApplyMinMax=off
      settings: SourceProductName=Simulink Real-Time  SourceProductBaseCode=XP  DataFormat=CANdb specified signals
  CAN Unpack4 : canmsglib/CAN Unpack  CANdbFile=D:\Work\02_LKA\LKAS\Documents\D53-PSA1CAN.dbc  MsgList=GW_32D_PSA1  MsgName=GW_32D_PSA1  MsgIDType=Standard (11-bit identifier)  MsgIdentifier=813  MsgLength=8  SignalInfo=ACCEL_LONGI_CALIB$12$12$2$2$1$0$2.000000e-02$-4.096000e+01$-4.096000e+01$4.092000e+01$#Brake_Pedal_Active$16$2$2$2$1$0$1$0$-Inf$Inf$#Braking_effort$9$1$2$2$1$0$1$0$-Inf$Inf$#ESC_ACC_Status$19$2$2$2$1$0$1$0$-Inf$Inf$#ESC_AEB_Status$10$2$2$2$1$0$1$0$-Inf$Inf$#Message_from_ESC_informing$23$1$2$2$1$0$1$0$-Inf$Inf$#UFC_to_ACC_dynamic_frame$56$4$2$2$1$0$1$0$-Inf$Inf$#Vehicle_Hold_Status$29$2$2$2$1$0$1$0$-Inf$Inf$#Vehicle_detected_as_stationary$21$1$2$2$1$0$1$0$-Inf$Inf$#YawRate_Raw$44$12$2$2$1$0$8.000000e-02$-1.638400e+02$-1.638400e+02$1.636800e+02$#bits_compute_counter_for_UCbrake$60$4$2$2$1$0$1$0$0$15$#  NSignals=11  IDPort=off  TimestampPort=off  ErrorPort=off  RemotePort=off  LengthPort=off  StatusPort=off  StartBits=str2num('[int32(12);int32(16);int32(9);int32(19);int32(10);int32(23);int32(56);int32(29);int32(21);int32(44);int32(60)]')  SignalSizes=str2num('[int32(12);int32(2);int32(1);int32(2);int32(2);int32(1);int32(4);int32(2);int32(1);int32(12);int32(4)]')  ByteOrders=str2num('[int32(2);int32(2);int32(2);int32(2);int32(2);int32(2);int32(2);int32(2);int32(2);int32(2);int32(2)]')  DataTypes=str2num('[int32(2);int32(2);int32(2);int32(2);int32(2);int32(2);int32(2);int32(2);int32(2);int32(2);int32(2)]')  MultiplexTypes=str2num('[int32(1);int32(1);int32(1);int32(1);int32(1);int32(1);int32(1);int32(1);int32(1);int32(1);int32(1)]')  MultiplexValues=str2num('[double(0);double(0);double(0);double(0);double(0);double(0);double(0);double(0);double(0);double(0);double(0)]')  Factors=str2num('[double(2.000000e-02);double(1);double(1);double(1);double(1);double(1);double(1);double(1);double(1);double(8.000000e-02);double(1)]')  Offsets=str2num('[double(-4.096000e+01);double(0);double(0);double(0);double(0);double(0);double(0);double(0);double(0);double(-1.638400e+02);double(0)]')  Minimums=str2num('[double(-4.096000e+01);double(-Inf);double(-Inf);double(-Inf);double(-Inf);double(-Inf);double(-Inf);double(-Inf);double(-Inf);double(-1.638400e+02);double(0)]')  Maximums=str2num('[double(4.092000e+01);double(Inf);double(Inf);double(Inf);double(Inf);double(Inf);double(Inf);double(Inf);double(Inf);double(1.636800e+02);double(15)]')  ApplyMinMax=off
      settings: SourceProductName=Simulink Real-Time  SourceProductBaseCode=XP  DataFormat=CANdb specified signals
  CAN_Receive4 : S-Function  FunctionName=CAN_Rec_P  Parameters=uint8(Module-1),uint32(ID),uint8(Frameformat-1),uint8(Newflag),uint8(FIFO),double(sampletime)  SFunctionDeploymentMode=off  EnableBusSupport=off  mask(CAN_receive){Module=CAN_1, ID=813, Frameformat=Standard (11-bit identifier), Newflag=off, FIFO=off, sampletime=0.02}
      mask prompts: Module "CAN Port:"; ID "CAN Frame ID:"; Frameformat "CAN Frame Format:"; FIFO "Overflow flag"
      mask init:
      | maskdisplay = canrecicon(Module,ID,Frameformat,Newflag,FIFO);
      | set_param(gcb, 'MaskDisplay', maskdisplay);
      mask TypeOptions Module: CAN_0 | CAN_1 | CAN_2 | CAN_3
      mask TypeOptions Frameformat: Standard (11-bit identifier) | Extended (29-bit identifier)
      mask Display: color('blue');text(0.98,0.9,'MPC5675K','horizontalAlignment','right');color('black');text(0.5,0.6,'FlexCAN_1 Receive','horizontalAlignment','center');text(0.5,0.35,'Standard ID:813','horizontalAlignment','center');port_label('output',1,'CAN_Msg');
  Data Type Conversion{1..5,11} (6 alike) : DataTypeConversion  OutDataTypeStr=single
  Data Type Conversion53 : DataTypeConversion  OutDataTypeStr=uint8
  Ground : Ground
  Ground1 : Ground
  Ground2 : Ground
  Rate Transition{,1..5,7} (7 alike) : RateTransition  OutPortSampleTime=0.01
  Terminator{,1..14} (15 alike) : Terminator
  bsVehMovInfo : Outport
  wires:
  CAN Unpack4/1 -> Rate Transition/1
  CAN Unpack/3 -> Rate Transition3/1
  CAN Unpack1/4 -> Rate Transition4/1
  Data Type Conversion2/1 -> Bus Creator9/3  "ESC_YawRate"
  Ground1/1 -> Bus Creator9/4  "ESC_YawRate_Valid"
  Rate Transition3/1 -> Data Type Conversion3/1
  CAN Unpack4/6 -> Terminator7/1
  CAN Unpack/1 -> Terminator2/1
  Rate Transition2/1 -> Data Type Conversion2/1
  Rate Transition7/1 -> Data Type Conversion5/1
  CAN Recv (CANRx])/1 -> CAN Unpack/1
  CAN Unpack1/3 -> Rate Transition7/1
  Data Type Conversion4/1 -> Bus Creator9/5  "ESC_UnYawRate"
  Data Type Conversion11/1 -> Bus Creator9/7  "ESC_LonAcc"
  CAN Unpack/4 -> Rate Transition1/1
  Data Type Conversion53/1 -> Bus Creator9/10  "ESC_VehSpd_Valid"
  Data Type Conversion3/1 -> Bus Creator9/1  "ESC_LatAcc"
  Rate Transition4/1 -> Data Type Conversion53/1
  Rate Transition5/1 -> Data Type Conversion4/1
  Ground2/1 -> Bus Creator9/2  "ESC_LatAcc_Valid"
  Rate Transition1/1 -> Data Type Conversion1/1
  CAN Unpack4/10 -> Rate Transition5/1
  Data Type Conversion1/1 -> Bus Creator9/9  "ESC_Brake_Press"
  CAN Unpack/5 -> Rate Transition2/1
  Rate Transition/1 -> Data Type Conversion11/1
  CAN Unpack4/11 -> Terminator11/1
  CAN Unpack/6 -> Terminator1/1
  Data Type Conversion5/1 -> Bus Creator9/6  "ESC_VehSpd"
  CAN Unpack/2 -> Terminator/1
  CAN Unpack4/4 -> Terminator5/1
  CAN_Receive4/1 -> CAN Unpack4/1
  CAN Unpack4/8 -> Terminator9/1
  CAN Unpack4/7 -> Terminator8/1
  CAN Unpack4/5 -> Terminator6/1
  CAN Unpack4/9 -> Terminator10/1
  CAN Unpack4/2 -> Terminator3/1
  CAN Unpack4/3 -> Terminator4/1
  Bus Creator9/1 -> bsVehMovInfo/1  "bsVehMovInfo"
  Ground/1 -> Bus Creator9/8  "ESC_LonAcc_Valid"
  CAN Recv (CANRx])1/1 -> CAN Unpack1/1
  CAN Unpack1/1 -> Terminator12/1
  CAN Unpack1/2 -> Terminator13/1
  CAN Unpack1/5 -> Terminator14/1

== system D53_LKAS_JLU_20200903_0931/SignalBusCreator/Subsystem9 ==
  Bus Creator4 : BusCreator  Inputs=2
  CAN Unpack1 : canmsglib/CAN Unpack  CANdbFile=D:\Work\02_LKA\LKAS\Documents\D53-PSA1CAN.dbc  MsgList=GW_228_PSA1  MsgName=GW_228_PSA1  MsgIDType=Standard (11-bit identifier)  MsgIdentifier=552  MsgLength=8  SignalInfo=EMS_Acceleration_pedal_position$16$8$2$2$1$0$5.000000e-01$0$0$100$#  NSignals=1  IDPort=off  TimestampPort=off  ErrorPort=off  RemotePort=off  LengthPort=off  StatusPort=off  StartBits=str2num('[int32(16)]')  SignalSizes=str2num('[int32(8)]')  ByteOrders=str2num('[int32(2)]')  DataTypes=str2num('[int32(2)]')  MultiplexTypes=str2num('[int32(1)]')  MultiplexValues=str2num('[double(0)]')  Factors=str2num('[double(5.000000e-01)]')  Offsets=str2num('[double(0)]')  Minimums=str2num('[double(0)]')  Maximums=str2num('[double(100)]')  ApplyMinMax=off
      settings: SourceProductName=Simulink Real-Time  SourceProductBaseCode=XP  DataFormat=CANdb specified signals
  CAN Unpack6 : canmsglib/CAN Unpack  CANdbFile=D:\Work\02_LKA\LKAS\Documents\D53-PSA1CAN.dbc  MsgList=GW_349_PSA1  MsgName=GW_349_PSA1  MsgIDType=Standard (11-bit identifier)  MsgIdentifier=841  MsgLength=8  SignalInfo=BV_dynamic_frame_checksum$52$4$2$2$1$0$1$0$-Inf$Inf$#TCU_AGB_Target_position$28$4$2$2$1$0$1$0$-Inf$Inf$#TCU_Gear_lever_position$24$4$2$2$1$0$1$0$-Inf$Inf$#bits_Compute_for_Gear_Box$48$4$2$2$1$0$1$0$0$15$#  NSignals=4  IDPort=off  TimestampPort=off  ErrorPort=off  RemotePort=off  LengthPort=off  StatusPort=off  StartBits=str2num('[int32(52);int32(28);int32(24);int32(48)]')  SignalSizes=str2num('[int32(4);int32(4);int32(4);int32(4)]')  ByteOrders=str2num('[int32(2);int32(2);int32(2);int32(2)]')  DataTypes=str2num('[int32(2);int32(2);int32(2);int32(2)]')  MultiplexTypes=str2num('[int32(1);int32(1);int32(1);int32(1)]')  MultiplexValues=str2num('[double(0);double(0);double(0);double(0)]')  Factors=str2num('[double(1);double(1);double(1);double(1)]')  Offsets=str2num('[double(0);double(0);double(0);double(0)]')  Minimums=str2num('[double(-Inf);double(-Inf);double(-Inf);double(0)]')  Maximums=str2num('[double(Inf);double(Inf);double(Inf);double(15)]')  ApplyMinMax=off
      settings: SourceProductName=Simulink Real-Time  SourceProductBaseCode=XP  DataFormat=CANdb specified signals
  CAN_Receive1 : S-Function  FunctionName=CAN_Rec_P  Parameters=uint8(Module-1),uint32(ID),uint8(Frameformat-1),uint8(Newflag),uint8(FIFO),double(sampletime)  SFunctionDeploymentMode=off  EnableBusSupport=off  mask(CAN_receive){Module=CAN_1, ID=552, Frameformat=Standard (11-bit identifier), Newflag=off, FIFO=off, sampletime=0.01}
      mask prompts: Module "CAN Port:"; ID "CAN Frame ID:"; Frameformat "CAN Frame Format:"; FIFO "Overflow flag"
      mask init:
      | maskdisplay = canrecicon(Module,ID,Frameformat,Newflag,FIFO);
      | set_param(gcb, 'MaskDisplay', maskdisplay);
      mask TypeOptions Module: CAN_0 | CAN_1 | CAN_2 | CAN_3
      mask TypeOptions Frameformat: Standard (11-bit identifier) | Extended (29-bit identifier)
      mask Display: color('blue');text(0.98,0.9,'MPC5675K','horizontalAlignment','right');color('black');text(0.5,0.6,'FlexCAN_1 Receive','horizontalAlignment','center');text(0.5,0.35,'Standard ID:552','horizontalAlignment','center');port_label('output',1,'CAN_Msg');
  CAN_Receive6 : S-Function  FunctionName=CAN_Rec_P  Parameters=uint8(Module-1),uint32(ID),uint8(Frameformat-1),uint8(Newflag),uint8(FIFO),double(sampletime)  SFunctionDeploymentMode=off  EnableBusSupport=off  mask(CAN_receive){Module=CAN_1, ID=841, Frameformat=Standard (11-bit identifier), Newflag=off, FIFO=off, sampletime=0.01}
      mask prompts: Module "CAN Port:"; ID "CAN Frame ID:"; Frameformat "CAN Frame Format:"; FIFO "Overflow flag"
      mask init:
      | maskdisplay = canrecicon(Module,ID,Frameformat,Newflag,FIFO);
      | set_param(gcb, 'MaskDisplay', maskdisplay);
      mask TypeOptions Module: CAN_0 | CAN_1 | CAN_2 | CAN_3
      mask TypeOptions Frameformat: Standard (11-bit identifier) | Extended (29-bit identifier)
      mask Display: color('blue');text(0.98,0.9,'MPC5675K','horizontalAlignment','right');color('black');text(0.5,0.6,'FlexCAN_1 Receive','horizontalAlignment','center');text(0.5,0.35,'Standard ID:841','horizontalAlignment','center');port_label('output',1,'CAN_Msg');
  Data Type Conversion1 : DataTypeConversion  OutDataTypeStr=uint8
  Data Type Conversion7 : DataTypeConversion  OutDataTypeStr=uint8
  Rate Transition1 : RateTransition  OutPortSampleTime=0.01
  Terminator : Terminator
  Terminator1 : Terminator
  Terminator2 : Terminator
  bsPTState : Outport
  wires:
  CAN Unpack6/3 -> Data Type Conversion7/1
  Bus Creator4/1 -> bsPTState/1  "bsPTState"
  CAN Unpack6/1 -> Terminator/1
  Data Type Conversion7/1 -> Bus Creator4/2  "TCU_ActualGear"
  CAN_Receive6/1 -> CAN Unpack6/1
  CAN Unpack6/4 -> Terminator1/1
  CAN_Receive1/1 -> CAN Unpack1/1
  CAN Unpack1/1 -> Rate Transition1/1
  Rate Transition1/1 -> Data Type Conversion1/1
  Data Type Conversion1/1 -> Bus Creator4/1  "AccPedal_Pos"
  CAN Unpack6/2 -> Terminator2/1

== system D53_LKAS_JLU_20200903_0931/LL/Human Machine Interface (HMI)/Subsystem ==
  LDW_STATE : Inport
  EPSInfo : Inport  Port=2
  Abs : Abs
  Bus Selector2 : BusSelector  OutputSignals=EPS_LKA_State,EPS_SW_Trq
  Compare1 : simulink/Logic and Bit Operations/Compare To Constant  relop===  const=3  OutDataTypeStr=boolean
  Compare2 : simulink/Logic and Bit Operations/Compare To Constant  relop===  const=3  OutDataTypeStr=boolean
  Compare3 : simulink/Logic and Bit Operations/Compare To Constant  relop===  const=1  OutDataTypeStr=boolean
  Compare4 : simulink/Logic and Bit Operations/Compare To Constant  relop===  const=3  OutDataTypeStr=boolean
  Compare5 : simulink/Logic and Bit Operations/Compare To Constant  relop===  const=4  OutDataTypeStr=boolean
  Compare6 : simulink/Logic and Bit Operations/Compare To Constant  relop===  const=5  OutDataTypeStr=boolean
  Constant : Constant  Value=0.25  OutDataTypeStr=single
  Constant1 : Constant  Value=0.5  OutDataTypeStr=single
  Count 10s : Subsystem
  Count 15s : Subsystem
  Logical Operator2 : Logic  AllPortsSameDT=off  OutDataTypeStr=boolean
  Logical Operator3 : Logic  Operator=OR  Inputs=5  AllPortsSameDT=off  OutDataTypeStr=boolean
  Relational Operator : RelationalOperator  Operator=<=  OutDataTypeStr=boolean  RndMeth=Nearest
  Switch : Switch  Criteria=u2 > Threshold
  HandsOff10s : Outport
  HandsOff15s : Outport  Port=2
  wires:
  Abs/1 -> Relational Operator/1
  Compare6/1 -> Logical Operator3/1
  Compare5/1 -> Logical Operator3/2
  Compare4/1 -> Logical Operator3/3
  LDW_STATE/1 -> Compare5/1, Compare6/1, Compare4/1
  Count 15s/1(Out) -> HandsOff15s/1
  Relational Operator/1 -> Logical Operator2/2
  Constant1/1 -> Switch/1
  Logical Operator3/1 -> Logical Operator2/1
  Logical Operator2/1 -> Count 10s/Enable, Count 15s/Enable
  Bus Selector2/2 -> Abs/1  "<EPS_SW_Trq>"
  Compare1/1 -> Switch/2
  Switch/1 -> Relational Operator/2
  EPSInfo/1 -> Bus Selector2/1
  Constant/1 -> Switch/3
  Bus Selector2/1 -> Compare2/1, Compare3/1, Compare1/1  "<EPS_LKA_State>"
  Compare2/1 -> Logical Operator3/4
  Compare3/1 -> Logical Operator3/5
  Count 10s/1(Out) -> HandsOff10s/1

== system D53_LKAS_JLU_20200903_0931/LL/LL Inputs Mapping/bsBCMInfo ==
  bsBCMInfoIn : Inport
  Bus Creator1 : BusCreator  Inputs=3
  Bus Selector1 : BusSelector  OutputSignals=BCM_Double_Light,BCM_Left_Light,BCM_Right_Light
  bsBCMInfoOut : Outport
  wires:
  bsBCMInfoIn/1 -> Bus Selector1/1
  Bus Selector1/1 -> Bus Creator1/1  "<BCM_Double_Light>"
  Bus Creator1/1 -> bsBCMInfoOut/1
  Bus Selector1/2 -> Bus Creator1/2  "<BCM_Left_Light>"
  Bus Selector1/3 -> Bus Creator1/3  "<BCM_Right_Light>"

== system D53_LKAS_JLU_20200903_0931/LL/LL Inputs Mapping/bsEPSInfo ==
  bsEPSInfoIn : Inport
  Bus Creator4 : BusCreator  Inputs=9
  Bus Selector1 : BusSelector  OutputSignals=EPS_LKA_State,EPS_SW_Trq,EPS_Error_State,EPS_Trq_State,SAS_Clb_State,SAS_Trim_State,EPS_TrqLim_State,EPS_LKA_Current,EPS_SWHold_State
  bsEPSInfoOut : Outport
  wires:
  bsEPSInfoIn/1 -> Bus Selector1/1
  Bus Selector1/2 -> Bus Creator4/2  "<EPS_SW_Trq>"
  Bus Selector1/1 -> Bus Creator4/1  "<EPS_LKA_State>"
  Bus Creator4/1 -> bsEPSInfoOut/1
  Bus Selector1/3 -> Bus Creator4/3  "<EPS_Error_State>"
  Bus Selector1/4 -> Bus Creator4/4  "<EPS_Trq_State>"
  Bus Selector1/5 -> Bus Creator4/5  "<SAS_Clb_State>"
  Bus Selector1/6 -> Bus Creator4/6  "<SAS_Trim_State>"
  Bus Selector1/7 -> Bus Creator4/7  "<EPS_TrqLim_State>"
  Bus Selector1/8 -> Bus Creator4/8  "<EPS_LKA_Current>"
  Bus Selector1/9 -> Bus Creator4/9  "<EPS_SWHold_State>"
